simulink model "die_hard_3"  (R2019b)
settings: Solver=FixedStepDiscrete  StartTime=0.0  StopTime=100000  FixedStep=1  RelTol=1e-3
values from neighbouring files (symbols this model uses):
  BIG = int32(5)    [die_hard_3_init.m]
  QUICK_TIME = int32(4)    [die_hard_3_init.m]
  SMALL = int32(3)    [die_hard_3_init.m]
  TARGET = int32(4)    [die_hard_3_init.m]
undefined symbols (not defined in the file or in its folder): t_action
libraries: common_lib x3
settings Model: Creator=F074018  LastModifiedBy=F074018
settings DataIOCC: ReturnWorkspaceOutputs=off
settings DebuggingCC: InheritedTsInSrcMsg=none  ArithmeticOperatorsInVariantConditions=warning
settings SFSimCC: CustomCodeUndefinedFunction=UseInterfaceOnly
settings ConfigComp: DVMode=PropertyProving  DVTestSuiteOptimization=Auto  DVDetectOutOfBounds=on

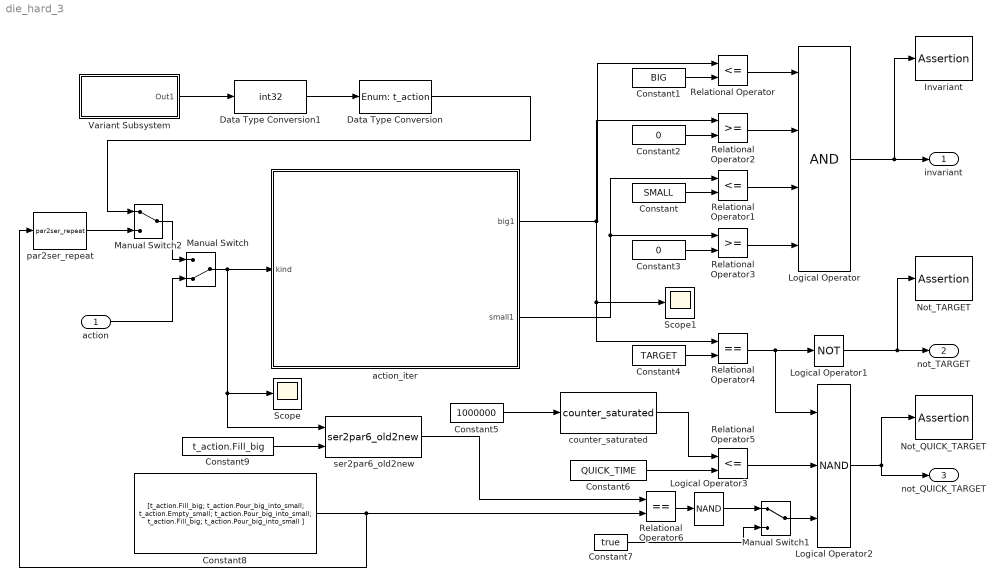
== system die_hard_3 ==
  action : Inport  OutDataTypeStr=Enum: t_action
      settings: AttributesFormatString=OutDataTypeStr=%<OutDataTypeStr>
  Constant : Constant  Value=SMALL  OutDataTypeStr=int32
  Constant1 : Constant  Value=BIG  OutDataTypeStr=int32
  Constant2 : Constant  Value=0  OutDataTypeStr=int32
  Constant3 : Constant  Value=0  OutDataTypeStr=int32
  Constant4 : Constant  Value=TARGET  OutDataTypeStr=int32
  Constant5 : Constant  Value=1000000  OutDataTypeStr=int32
  Constant6 : Constant  Value=QUICK_TIME  OutDataTypeStr=int32
  Constant7 : Constant  Value=true
  Constant8 : Constant  Value=[t_action.Fill_big; t_action.Pour_big_into_small; t_action.Empty_small; t_action.Pour_big_into_small; t_action.Fill_big; t_action.Pour_big_into_small ]  VectorParams1D=off  OutDataTypeStr=Enum: t_action
  Constant9 : Constant  Value=t_action.Fill_big  OutDataTypeStr=Enum: t_action
  Data Type Conversion : DataTypeConversion  OutDataTypeStr=Enum: t_action
      settings: AttributesFormatString=OutDataTypeStr=%<OutDataTypeStr>
  Data Type Conversion1 : DataTypeConversion  OutDataTypeStr=int32  RndMeth=Round
      settings: AttributesFormatString=RndMeth=%<RndMeth>
  Invariant : Assertion
  Logical Operator : Logic  Inputs=4  IconShape=distinctive  AllPortsSameDT=off  OutDataTypeStr=boolean
  Logical Operator1 : Logic  Operator=NOT  IconShape=distinctive  AllPortsSameDT=off  OutDataTypeStr=boolean
  Logical Operator2 : Logic  Operator=NAND  Inputs=3  IconShape=distinctive  AllPortsSameDT=off  OutDataTypeStr=boolean
  Logical Operator3 : Logic  Operator=NAND  Inputs=1  IconShape=distinctive  OutDataTypeStr=boolean
  Manual Switch : ManualSwitch  CurrentSetting=0
  Manual Switch1 : ManualSwitch
  Manual Switch2 : ManualSwitch
  Not_QUICK_TARGET : Assertion  Enabled=off
  Not_TARGET : Assertion
  Relational Operator : RelationalOperator  Operator=<=  OutDataTypeStr=boolean  RndMeth=Simplest  InputSameDT=on
  Relational Operator1 : RelationalOperator  Operator=<=  OutDataTypeStr=boolean  RndMeth=Simplest  InputSameDT=on
  Relational Operator2 : RelationalOperator  OutDataTypeStr=boolean  RndMeth=Simplest  InputSameDT=on
  Relational Operator3 : RelationalOperator  OutDataTypeStr=boolean  RndMeth=Simplest  InputSameDT=on
  Relational Operator4 : RelationalOperator  Operator===  OutDataTypeStr=boolean  RndMeth=Simplest  InputSameDT=on
  Relational Operator5 : RelationalOperator  Operator=<=  OutDataTypeStr=boolean  RndMeth=Simplest  InputSameDT=on
  Relational Operator6 : RelationalOperator  Operator===  OutDataTypeStr=boolean  RndMeth=Simplest  InputSameDT=on
  Scope : Scope
  Scope1 : Scope
  Variant Subsystem : Subsystem  Variant=on
  action_iter : Subsystem
  counter_saturated : common_lib/counter_saturated  SystemSampleTime=-1  Latency=0  AutoFrameSizeCalculation=off
  par2ser_repeat : common_lib/par2ser_repeat  SystemSampleTime=-1  Latency=0  AutoFrameSizeCalculation=off
  ser2par6_old2new : common_lib/ser2par6_old2new  SystemSampleTime=-1  Latency=0  AutoFrameSizeCalculation=off
  invariant : Outport  VectorParamsAs1DForOutWhenUnconnected=off
  not_TARGET : Outport  Port=2  VectorParamsAs1DForOutWhenUnconnected=off
  not_QUICK_TARGET : Outport  Port=3  VectorParamsAs1DForOutWhenUnconnected=off
  wires:
  action_iter/1(big1) -> Scope1/1, Relational Operator4/1, Relational Operator2/1, Relational Operator/1
  action_iter/2(small1) -> Relational Operator3/1, Relational Operator1/1
  Constant1/1 -> Relational Operator/2
  Constant2/1 -> Relational Operator2/2
  Constant/1 -> Relational Operator1/2
  Constant3/1 -> Relational Operator3/2
  Constant4/1 -> Relational Operator4/2
  Relational Operator3/1 -> Logical Operator/4
  Relational Operator1/1 -> Logical Operator/3
  Relational Operator2/1 -> Logical Operator/2
  Relational Operator/1 -> Logical Operator/1
  Logical Operator/1 -> invariant/1, Invariant/1
  Variant Subsystem/1(Out1) -> Data Type Conversion1/1
  Data Type Conversion1/1 -> Data Type Conversion/1
  Manual Switch/1 -> Scope/1, ser2par6_old2new/1, action_iter/1(kind)
  action/1 -> Manual Switch/2
  Relational Operator4/1 -> Logical Operator2/1, Logical Operator1/1
  Logical Operator1/1 -> not_TARGET/1, Not_TARGET/1
  Constant5/1 -> counter_saturated/1
  counter_saturated/1 -> Relational Operator5/1
  Constant6/1 -> Relational Operator5/2
  Relational Operator5/1 -> Logical Operator2/2
  Logical Operator2/1 -> Not_QUICK_TARGET/1, not_QUICK_TARGET/1
  Manual Switch1/1 -> Logical Operator2/3
  Logical Operator3/1 -> Manual Switch1/1
  Constant7/1 -> Manual Switch1/2
  Relational Operator6/1 -> Logical Operator3/1
  ser2par6_old2new/1 -> Relational Operator6/1
  Constant8/1 -> par2ser_repeat/1, Relational Operator6/2
  Constant9/1 -> ser2par6_old2new/2
  Manual Switch2/1 -> Manual Switch/1
  Data Type Conversion/1 -> Manual Switch2/1
  par2ser_repeat/1 -> Manual Switch2/2

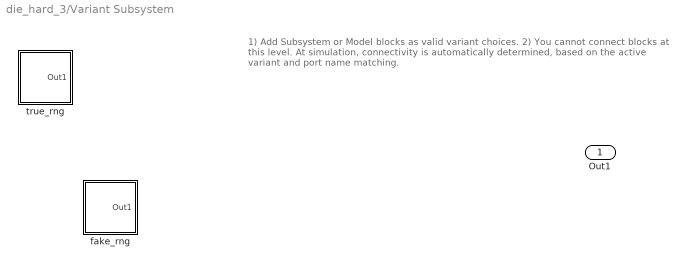
== system die_hard_3/Variant Subsystem ==
  note: 1) Add Subsystem or Model blocks as valid variant choices.
      | 2) You cannot connect blocks at this level. At simulation, connectivity is automatically
      | determined, based on the active variant and port name matching.
  fake_rng : Subsystem  VariantControl=variant_true_rng == false
  true_rng : Subsystem  VariantControl=(default)
  Out1 : Outport  VectorParamsAs1DForOutWhenUnconnected=off

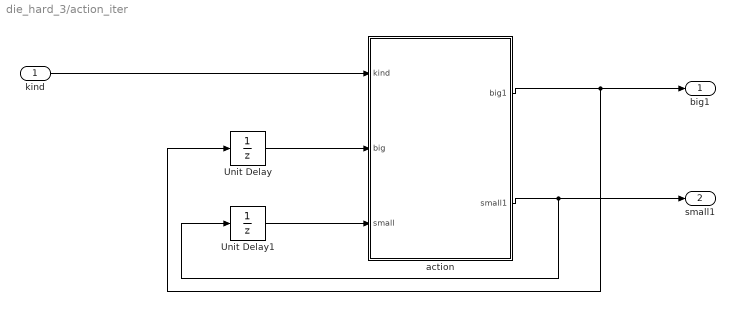
== system die_hard_3/action_iter ==
  kind : Inport  OutDataTypeStr=Enum: t_action
  Unit Delay : UnitDelay  InitialCondition=int32(0)  SampleTime=-1  HasFrameUpgradeWarning=on
      settings: AttributesFormatString=InitialCondition=%<InitialCondition>
  Unit Delay1 : UnitDelay  InitialCondition=int32(0)  SampleTime=-1  HasFrameUpgradeWarning=on
      settings: AttributesFormatString=InitialCondition=%<InitialCondition>
  action : Subsystem
  big1 : Outport  VectorParamsAs1DForOutWhenUnconnected=off
  small1 : Outport  Port=2  VectorParamsAs1DForOutWhenUnconnected=off
  wires:
  kind/1 -> action/1(kind)
  Unit Delay1/1 -> action/3(small)
  action/1(big1) -> Unit Delay/1, big1/1
  action/2(small1) -> Unit Delay1/1, small1/1
  Unit Delay/1 -> action/2(big)

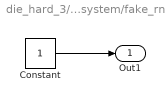
== system die_hard_3/Variant Subsystem/fake_rng ==
  Constant : Constant
  Out1 : Outport  VectorParamsAs1DForOutWhenUnconnected=off
  wires:
  Constant/1 -> Out1/1

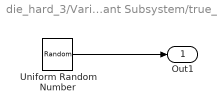
== system die_hard_3/Variant Subsystem/true_rng ==
  Uniform Random Number : UniformRandomNumber  Minimum=-0.5  Maximum=5.5
      settings: AttributesFormatString=|
      | Minimum=%<Minimum>
      | Maximum=%<Maximum>
  Out1 : Outport  VectorParamsAs1DForOutWhenUnconnected=off
  wires:
  Uniform Random Number/1 -> Out1/1

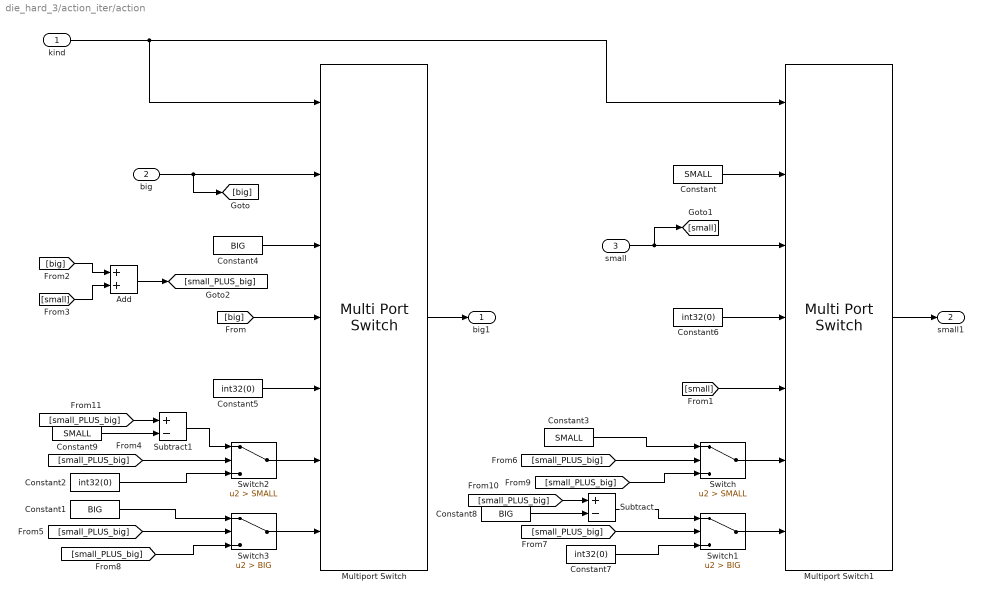
== system die_hard_3/action_iter/action ==
  kind : Inport  OutDataTypeStr=Enum: t_action
  big : Inport  Port=2  OutDataTypeStr=int32
  small : Inport  Port=3  OutDataTypeStr=int32
  Add : Sum
  Constant : Constant  Value=SMALL
  Constant1 : Constant  Value=BIG
  Constant{2,5..7} (4 alike) : Constant  Value=int32(0)
  Constant3 : Constant  Value=SMALL
  Constant4 : Constant  Value=BIG
  Constant8 : Constant  Value=BIG
  Constant9 : Constant  Value=SMALL
  Multiport Switch : MultiPortSwitch  DataPortOrder=Specify indices  Inputs=6  DataPortIndices={t_action.Fill_small, t_action.Fill_big, t_action.Empty_small, t_action.Empty_big, t_action.Pour_big_into_small, t_action.Pour_small_into_big}  DiagnosticForDefault=None  InputSameDT=on
  Multiport Switch1 : MultiPortSwitch  DataPortOrder=Specify indices  Inputs=6  DataPortIndices={t_action.Fill_small, t_action.Fill_big, t_action.Empty_small, t_action.Empty_big, t_action.Pour_big_into_small, t_action.Pour_small_into_big}  DiagnosticForDefault=None  InputSameDT=on
  Subtract : Sum  Inputs=+-
  Subtract1 : Sum  Inputs=+-
  Switch : Switch  Criteria=u2 > Threshold  Threshold=SMALL  InputSameDT=on
  Switch1 : Switch  Criteria=u2 > Threshold  Threshold=BIG  InputSameDT=on
  Switch2 : Switch  Criteria=u2 > Threshold  Threshold=SMALL  InputSameDT=on
  Switch3 : Switch  Criteria=u2 > Threshold  Threshold=BIG  InputSameDT=on
  big1 : Outport  VectorParamsAs1DForOutWhenUnconnected=off
  small1 : Outport  Port=2  VectorParamsAs1DForOutWhenUnconnected=off
  wires:
  Multiport Switch/1 -> big1/1
  kind/1 -> Multiport Switch/1, Multiport Switch1/1
  big/1 -> [big], Multiport Switch/2
  Multiport Switch1/1 -> small1/1
  Constant4/1 -> Multiport Switch/3
  Constant5/1 -> Multiport Switch/5
  Constant/1 -> Multiport Switch1/2
  small/1 -> [small], Multiport Switch1/3
  Constant6/1 -> Multiport Switch1/4
  [big] -> Multiport Switch/4
  [small] -> Multiport Switch1/5
  Switch/1 -> Multiport Switch1/6
  Switch1/1 -> Multiport Switch1/7
  Switch2/1 -> Multiport Switch/6
  Switch3/1 -> Multiport Switch/7
  [big] -> Add/1
  [small] -> Add/2
  Add/1 -> [small_PLUS_big]
  [small_PLUS_big] -> Switch2/2
  [small_PLUS_big] -> Switch3/2
  [small_PLUS_big] -> Switch/2
  [small_PLUS_big] -> Switch1/2
  Constant1/1 -> Switch3/1
  [small_PLUS_big] -> Switch3/3
  Constant2/1 -> Switch2/3
  Constant3/1 -> Switch/1
  [small_PLUS_big] -> Switch/3
  Constant7/1 -> Switch1/3
  Subtract/1 -> Switch1/1
  [small_PLUS_big] -> Subtract/1
  Constant8/1 -> Subtract/2
  Constant9/1 -> Subtract1/2
  [small_PLUS_big] -> Subtract1/1
  Subtract1/1 -> Switch2/1
